simulink model "MagLev_SMC"  (R2024b)
settings: Solver=VariableStepAuto  StartTime=0.0  StopTime=10.0  FixedStep=1e-5  RelTol=1e-3
undefined symbols (not defined in the file or in its folder): g, k, m
settings Model: Creator=98912  LastModifiedBy=98912
settings DataIOCC: SaveFormat=Array

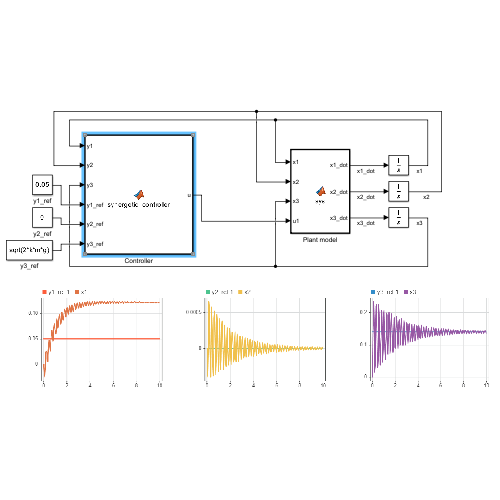
[thumbnail: Simulink's stored preview of the top-level diagram]
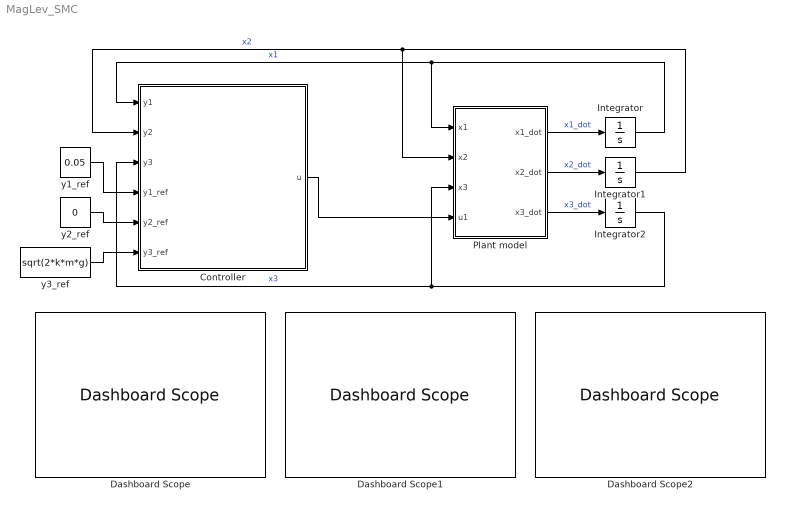
== system MagLev_SMC ==
  Controller : MATLAB Function  TreatAsAtomicUnit=on
  Dashboard Scope : DashboardScope
  Dashboard Scope1 : DashboardScope
  Dashboard Scope2 : DashboardScope
  Integrator : Integrator
  Integrator1 : Integrator
  Integrator2 : Integrator
  Plant model : MATLAB Function  TreatAsAtomicUnit=on
  y1_ref : Constant  Value=0.05
  y2_ref : Constant  Value=0
  y3_ref : Constant  Value=sqrt(2*k*m*g)
  wires:
  Plant model/1(x1_dot) -> Integrator/1  "x1_dot"
  Plant model/2(x2_dot) -> Integrator1/1  "x2_dot"
  Plant model/3(x3_dot) -> Integrator2/1  "x3_dot"
  Integrator/1 -> Controller/1(y1), Plant model/1(x1)  "x1"
  Integrator1/1 -> Plant model/2(x2), Controller/2(y2)  "x2"
  Integrator2/1 -> Controller/3(y3), Plant model/3(x3)  "x3"
  Controller/1(u) -> Plant model/4(u1)
  y1_ref/1 -> Controller/4(y1_ref)
  y3_ref/1 -> Controller/6(y3_ref)
  y2_ref/1 -> Controller/5(y2_ref)

== matlab function MagLev_SMC/Controller ==
  data: y1 input; u output; y2 input; y3 input; y1_ref input; y2_ref input; y3_ref input
function u = synergetic_controller(y1, y2, y3, y1_ref, y2_ref, y3_ref)
% Implements the Synergetic Controller from Equation (73) of the paper.
%
% Inputs from Simulink:
% y1: current position (state x1)
% y2: current momentum (state x2)
% y3: current flux (state x3)
% y1_ref: desired position reference
% y2_ref: desired momentum reference (usually 0)
% y3_ref: desired flux reference (can be a constant or calculated)

% --- System and Controller Parameters ---
% These should match your plant model and the paper's Table 2
% System Parameters
m = 1.0/1000; % Mass of the ball in kg (1.00g)
g = 9.8;      % Gravitational constant
k = 1.0;      % Coil constant
R = 1.0;      % Resistance of the coil

% Controller Gains (from paper's Table 2 for Synergetic Control)
w0 = 6;
w1 = 6.03;
w2 = 0.5;
T  = 0.5;

% --- Controller Logic ---

% 1. Calculate errors (matches paper's e0, e1, e2)
e0 = y1 - y1_ref;
e1 = y2 - y2_ref;
e2 = y3 - y3_ref;

% 2. Calculate the macro-variable Omega (matches Eq. 66)
Omega = w0*e0 + w1*e1 + w2*e2;

% 3. Implement the final control law u from Equation (73)
% This equation is derived by solving for 'u' to make the system stable.
% u = (1/w2) * [ (w0*y1_ref + w1*y2_ref + w2*y3_ref - Omega/T) + ...
%                 w1*m*g - w0*y2/m - w1*y3^2/(2*k) + w2*R*(1-y1)*y3/k ]

term1 = w0*y1_ref + w1*y2_ref + w2*y3_ref - Omega/T;
term2 = w1*m*g;
term3 = -w0 * (y2/m);
term4 = -w1 * (y3^2 / (2*k));
term5 = w2 * R * (1-y1) * y3 / k;

u = (1/w2) * (term1 + term2 + term3 + term4 + term5);

end

== matlab function MagLev_SMC/Plant model ==
  data: x1 input; x1_dot output; x2 input; x3 input; u1 input; x2_dot output; x3_dot output
function [x1_dot, x2_dot, x3_dot] = sys(x1, x2, x3, u1)
    % System Parameters from Paper Table 1
    m = 1.0/1000; % Mass of the ball in kg (1.00g)
    g = 9.8;      % Gravitational constant
    k = 1.0;      % Coil constant
    R = 1.0;      % Resistance of the coil

    % Differential Equations from Paper (Eq. 19, 20, 21)
    x1_dot = x2 / m;
    x2_dot = (x3^2) / (2*k) - m*g;
    x3_dot = -R*(1-x1)*x3/k + u1;
end
